simulink model "Bloques1"  (R2021b)
settings: Solver=VariableStepAuto  StartTime=0.0  StopTime=10.0  RelTol=1e-3
settings Model: Creator=parra  LastModifiedBy=parra

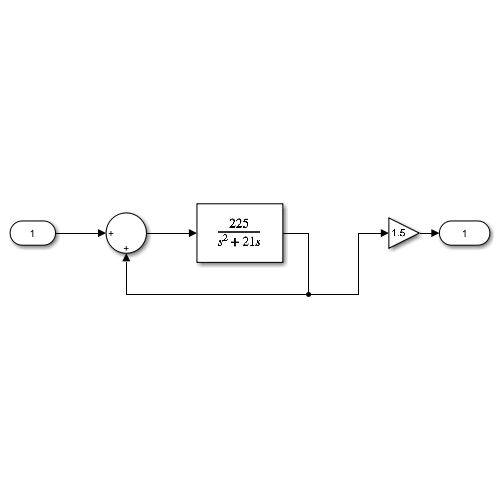
[thumbnail: Simulink's stored preview of the top-level diagram]
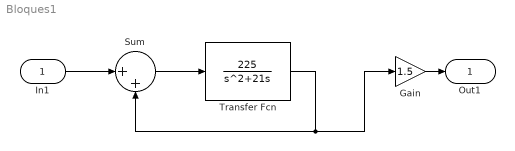
== system Bloques1 ==
  In1 : Inport
  Gain : Gain  Gain=1.5
  Sum : Sum  Inputs=|++
  Transfer Fcn : TransferFcn  Numerator=[225]  Denominator=[ 1 21 0]
  Out1 : Outport
  wires:
  In1/1 -> Sum/1
  Sum/1 -> Transfer Fcn/1
  Transfer Fcn/1 -> Gain/1, Sum/2
  Gain/1 -> Out1/1
